simulink model "Getriebe"  (Simulink 7.1)
settings: Solver=ode45  StartTime=0.0  StopTime=10.0  RelTol=1e-3
undefined symbols (not defined in the file): c, d, i, Jc, wirk
settings Model: Creator=dep19025415  LastModifiedBy=dep19025415

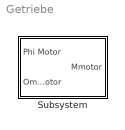
== system Getriebe ==
  Subsystem : Subsystem

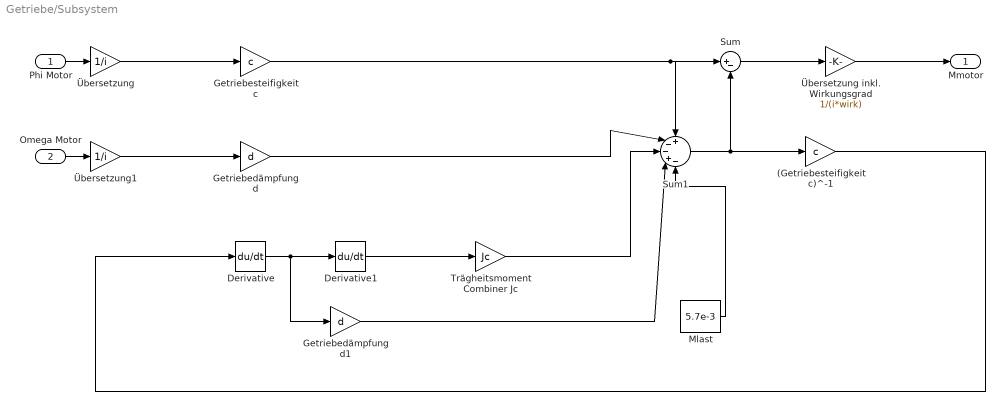
== system Getriebe/Subsystem ==
  Phi Motor : Inport
  Omega Motor : Inport  Port=2
  (Getriebesteifigkeit c)^-1 : Gain  Gain=c  ParameterDataType=sfix(16)  ParameterScaling=2^0  OutDataType=sfix(16)  OutScaling=2^0
  Derivative : Derivative
  Derivative1 : Derivative
  Getriebedämpfung d : Gain  Gain=d  ParameterDataType=sfix(16)  ParameterScaling=2^0  OutDataType=sfix(16)  OutScaling=2^0
  Getriebedämpfung d1 : Gain  Gain=d  ParameterDataType=sfix(16)  ParameterScaling=2^0  OutDataType=sfix(16)  OutScaling=2^0
  Getriebesteifigkeit c : Gain  Gain=c  ParameterDataType=sfix(16)  ParameterScaling=2^0  OutDataType=sfix(16)  OutScaling=2^0
  Mlast : Constant  Value=5.7e-3  OutDataType=sfix(16)  OutScaling=2^0
  Sum : Sum  Inputs=|+-  OutDataType=sfix(16)  OutScaling=2^0
  Sum1 : Sum  Inputs=+--+-  OutDataType=sfix(16)  OutScaling=2^0
  Trägheitsmoment Combiner Jc : Gain  Gain=Jc  ParameterDataType=sfix(16)  ParameterScaling=2^0  OutDataType=sfix(16)  OutScaling=2^0
  Übersetzung : Gain  Gain=1/i  ParameterDataType=sfix(16)  ParameterScaling=2^0  OutDataType=sfix(16)  OutScaling=2^0
  Übersetzung inkl. Wirkungsgrad : Gain  Gain=1/(i*wirk)  ParameterDataType=sfix(16)  ParameterScaling=2^0  OutDataType=sfix(16)  OutScaling=2^0
  Übersetzung1 : Gain  Gain=1/i  ParameterDataType=sfix(16)  ParameterScaling=2^0  OutDataType=sfix(16)  OutScaling=2^0
  Mmotor : Outport
  wires:
  Übersetzung/1 -> Getriebesteifigkeit c/1
  Übersetzung1/1 -> Getriebedämpfung d/1
  Getriebesteifigkeit c/1 -> Sum/1, Sum1/1
  Getriebedämpfung d/1 -> Sum1/2
  Sum1/1 -> (Getriebesteifigkeit c)^-1/1, Sum/2
  (Getriebesteifigkeit c)^-1/1 -> Derivative/1
  Derivative/1 -> Derivative1/1, Getriebedämpfung d1/1
  Derivative1/1 -> Trägheitsmoment Combiner Jc/1
  Trägheitsmoment Combiner Jc/1 -> Sum1/3
  Getriebedämpfung d1/1 -> Sum1/4
  Mlast/1 -> Sum1/5
  Sum/1 -> Übersetzung inkl. Wirkungsgrad/1
  Phi Motor/1 -> Übersetzung/1
  Übersetzung inkl. Wirkungsgrad/1 -> Mmotor/1
  Omega Motor/1 -> Übersetzung1/1
